simulink model "dsb"  (Simulink 7.1)
settings: Solver=ode45  StartTime=0.0  StopTime=1.0  RelTol=1e-3
undefined symbols (not defined in the file): ac, fc, fs, ka
libraries: dsparch4 x1
settings Model: Creator=08080002701  LastModifiedBy=08080002701

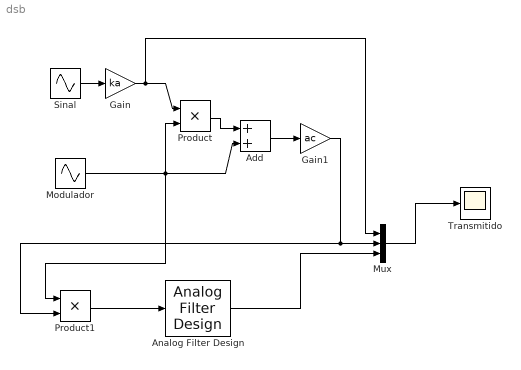
== system dsb ==
  Add : Sum  OutDataType=sfix(16)  OutScaling=2^-10
  Analog Filter Design : dsparch4/Analog Filter Design  method=Butterworth  filttype=Lowpass  N=8  Wlo=fc  Whi=80  Rp=2  Rs=40
  Gain : Gain  Gain=ka  ParameterDataType=sfix(16)  ParameterScaling=2^0  OutDataType=sfix(16)  OutScaling=2^0
  Gain1 : Gain  Gain=ac  ParameterDataType=sfix(16)  ParameterScaling=2^0  OutDataType=sfix(16)  OutScaling=2^0
  Modulador : Sin  Frequency=2*pi*fc  SampleTime=0
  Mux : Mux  Inputs=3
  Product : Product  OutDataType=sfix(16)  OutScaling=2^0  RndMeth=Zero
  Product1 : Product  OutDataType=sfix(16)  OutScaling=2^0  RndMeth=Zero
  Sinal : Sin  Frequency=2*pi*fs  SampleTime=0
  Transmitido : Scope
      settings: TimeRange=1  YMin=-1.5  YMax=1.5  DataFormat=Array  SampleInput=on  SampleTime=0.001
  wires:
  Sinal/1 -> Gain/1
  Modulador/1 -> Product/2, Add/2, Product1/1
  Gain/1 -> Product/1, Mux/1
  Product/1 -> Add/1
  Add/1 -> Gain1/1
  Gain1/1 -> Product1/2, Mux/2
  Product1/1 -> Analog Filter Design/1
  Mux/1 -> Transmitido/1
  Analog Filter Design/1 -> Mux/3
